simulink model "SympatheticCurrent_Parallel"  (R2015a)
settings: Solver=ode45  StartTime=0.0  StopTime=2  RelTol=1e-4
undefined symbols (not defined in the file or in its folder): D11, Delta
libraries: powerlib x15
settings Model: Creator=baishuhua  LastModifiedBy=baishuhua
settings DebuggingCC: AlgebraicLoopMsg=none

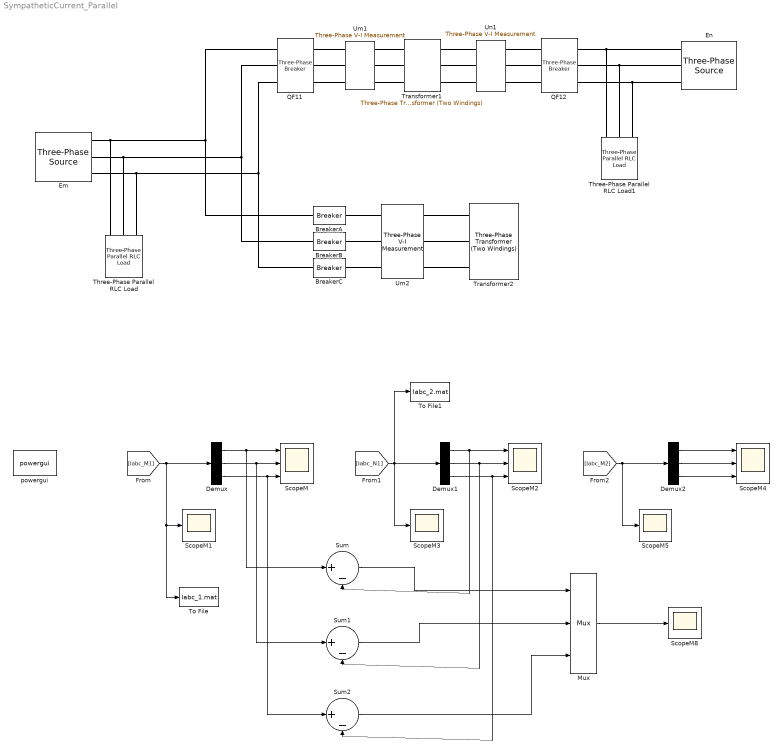
== system SympatheticCurrent_Parallel ==
  BreakerA : powerlib/Elements/Breaker  InitialState=0  SwitchingTimes=[1.1 2]  External=off  BreakerResistance=0.01  SnubberResistance=1e6  SnubberCapacitance=inf  Measurements=None  MoreParameters=on  NoBreakLoop=off
  BreakerB : powerlib/Elements/Breaker  InitialState=0  SwitchingTimes=[1.2 2]  External=off  BreakerResistance=0.01  SnubberResistance=1e6  SnubberCapacitance=inf  Measurements=None  MoreParameters=on  NoBreakLoop=off
  BreakerC : powerlib/Elements/Breaker  InitialState=0  SwitchingTimes=[1.3 2]  External=off  BreakerResistance=0.01  SnubberResistance=1e6  SnubberCapacitance=inf  Measurements=None  MoreParameters=on  NoBreakLoop=off
  Demux : Demux  Outputs=3
  Demux1 : Demux  Outputs=3
  Demux2 : Demux  Outputs=3
  Em : powerlib/Electrical Sources/Three-Phase Source  Voltage=35e3  PhaseAngle=180  Frequency=50  InternalConnection=Yg  SpecifyImpedance=off  Resistance=2.8929  Inductance=16.58e-3  ShortCircuitLevel=100e6  BaseVoltage=35e3  XRratio=7  BusType=swing  Pref=0  Qref=0  Qmin=-inf  Qmax=inf
  En : powerlib/Electrical Sources/Three-Phase Source  Voltage=220e3  PhaseAngle=0  Frequency=50  InternalConnection=Yg  SpecifyImpedance=off  Resistance=0.8929  Inductance=16.58e-3  ShortCircuitLevel=100e6  BaseVoltage=220e3  XRratio=7  BusType=swing  Pref=0  Qref=0  Qmin=-inf  Qmax=inf
  Mux : Mux  Inputs=3
  QF11 : powerlib/Elements/Three-Phase Breaker  InitialState=closed  SwitchA=on  SwitchB=on  SwitchC=on  SwitchTimes="[10  20]"  External=off  BreakerResistance=0.01  SnubberResistance=1e6  SnubberCapacitance=inf  Measurements=None
  QF12 : powerlib/Elements/Three-Phase Breaker  InitialState=open  SwitchA=on  SwitchB=on  SwitchC=on  SwitchTimes=[3 10]  External=off  BreakerResistance=0.01  SnubberResistance=1e6  SnubberCapacitance=inf  Measurements=None
  ScopeM : Scope  NumInputPorts=3
      settings: ShowLegends=on  TimeRange=2  YMin=-500~-4000~-1750  YMax=4000~500~250  SampleInput=on
  ScopeM{1,3,5,8} (4 alike) : Scope
      ScopeM1 settings: ShowLegends=on  TimeRange=5  YMin=-500  YMax=4000  SampleInput=on
      ScopeM3 settings: ShowLegends=on  TimeRange=5  YMin=-500  YMax=4000  SaveName=ScopeData3  SampleInput=on
      ScopeM5 settings: ShowLegends=on  TimeRange=5  YMin=-500  YMax=4000  SaveName=ScopeData5  SampleInput=on
      ScopeM8 settings: ShowLegends=on  TimeRange=5  YMin=-500  YMax=4000  SaveName=ScopeData8  SampleInput=on
  ScopeM2 : Scope  NumInputPorts=3
      settings: ShowLegends=on  TimeRange=1  YMin=-500~-4000~-1750  YMax=4000~500~250  SaveName=ScopeData2  SampleInput=on
  ScopeM4 : Scope  NumInputPorts=3
      settings: ShowLegends=on  TimeRange=10  YMin=-500~-4000~-1750  YMax=4000~500~250  SaveName=ScopeData4  SampleInput=on
  Sum : Sum  Inputs=|+-
  Sum1 : Sum  Inputs=|+-
  Sum2 : Sum  Inputs=|+-
  Three-Phase Parallel RLC Load : powerlib/Elements/Three-Phase Parallel RLC Load  LConnTagsString=A|B|C  Configuration=Y (grounded)  NominalVoltage=35e3  NominalFrequency=50  ActivePower=10e3  InductivePower=100  CapacitivePower=100  Measurements=None  LoadType=constant PQ
  Three-Phase Parallel RLC Load1 : powerlib/Elements/Three-Phase Parallel RLC Load  LConnTagsString=A|B|C  Configuration=Y (grounded)  NominalVoltage=220e3  NominalFrequency=50  ActivePower=10e3  InductivePower=100  CapacitivePower=100  Measurements=None  LoadType=constant PQ
  To File : ToFile  Filename=Iabc_1.mat  MatrixName=Iabc_1  SaveFormat=Timeseries
  To File1 : ToFile  Filename=Iabc_2.mat  MatrixName=Iabc_2  SaveFormat=Timeseries
  Transformer1 : powerlib/Elements/Three-Phase Transformer (Two Windings)  Winding1Connection=Delta (D11)  Winding2Connection=Delta (D11)  CoreType=Three single-phase transformers  SetSaturation=on  Hysteresis=off  DataFile='hysteresis'  SetInitialFlux=on  Measurements=None  UNITS=pu  NominalPower=[ 300e6 , 50 ]  Winding1=[ 35e3 , 0.002 , 0.08 ]  Winding2=[ 220e3 , 0.002 , 0.08 ]  Rm=500  Lm=500  L0=0.5  Saturation=[ 0,0 ; 0.0024,1.2 ; 1.0,1.52 ]  InitialFluxes=[0.5 0 0]  MoreParameters=off  BreakLoop=off  DataType=off  TransfoNumber=1
  Transformer2 : powerlib/Elements/Three-Phase Transformer (Two Windings)  Winding1Connection=Delta (D11)  Winding2Connection=Delta (D11)  CoreType=Three single-phase transformers  SetSaturation=on  Hysteresis=off  DataFile='hysteresis'  SetInitialFlux=on  Measurements=None  UNITS=pu  NominalPower=[ 300e6 , 50 ]  Winding1=[ 35e3 , 0.002 , 0.08 ]  Winding2=[ 220e3 , 0.002 , 0.08 ]  Rm=500  Lm=500  L0=0.5  Saturation=[ 0,0 ; 0.0024,1.2 ; 1.0,1.52 ]  InitialFluxes=[0.7 -0.7 -0.7]  MoreParameters=off  BreakLoop=off  DataType=off  TransfoNumber=1
  Um1 : powerlib/Measurements/Three-Phase V-I Measurement  VoltageMeasurement=no  SetLabelV=on  LabelV=Vabc_M  Vpu=off  VpuLL=off  CurrentMeasurement=yes  SetLabelI=on  LabelI=Iabc_M1  Ipu=on  Pbase=300e6  Vbase=35e3  OutputType=Complex  PhasorSimulation=off  PSBequivalent=0
  Um2 : powerlib/Measurements/Three-Phase V-I Measurement  VoltageMeasurement=no  SetLabelV=on  LabelV=Vabc_M  Vpu=off  VpuLL=off  CurrentMeasurement=yes  SetLabelI=on  LabelI=Iabc_M2  Ipu=on  Pbase=300e6  Vbase=35e3  OutputType=Complex  PhasorSimulation=off  PSBequivalent=0
  Un1 : powerlib/Measurements/Three-Phase V-I Measurement  VoltageMeasurement=no  SetLabelV=on  LabelV=Vabc_N  Vpu=off  VpuLL=off  CurrentMeasurement=yes  SetLabelI=on  LabelI=Iabc_N1  Ipu=on  Pbase=300e6  Vbase=220e3  OutputType=Complex  PhasorSimulation=off  PSBequivalent=0
  powergui : powerlib/powergui  Priority=1  SimulationMode=Discrete  SolverType=Tustin/Backward Euler (TBE)  SampleTime=1e-4  frequency=60  SPID=off  DisableSnubberDevices=off  DisableRonSwitches=off  DisableVfSwitches=off  SwTol=0  DisplayEquations=off  Interpol=off  methode=off  Ts=100  FunctionMessages=off  echomessages=off  HookPort=off  EnableUseOfTLC=off  x0status=blocks  frequencyindice=0  Pbase=100e6  ErrMax=1e-4  Iterations=50  UnitsV=kV  UnitsW=MW  buscounter=0  RestoreLinks=warning  ResistiveCurrentMeasurement=off  Frange=[0:2:500]  Ylog=off  Xlog=on  ShowGrid=off  save=off  variable=ZData  structure=0  ZoomFFT=off  StartTime=0.0  cycles=1  DisplayStyle=1  fundamental=60  FreqAxis=off  MaxFrequency=1000  frequencyindicesteady=1  RmsSteady=1  display=off
  wires:
  [Iabc_M1] -> To File/1, ScopeM1/1, Demux/1
  Demux/1 -> Sum/1, ScopeM/1
  Demux/2 -> ScopeM/2, Sum1/1
  Demux/3 -> ScopeM/3, Sum2/1
  [Iabc_N1] -> To File1/1, ScopeM3/1, Demux1/1
  Demux1/1 -> ScopeM2/1, Sum/2
  Demux1/2 -> ScopeM2/2, Sum1/2
  Demux1/3 -> Sum2/2, ScopeM2/3
  [Iabc_M2] -> ScopeM5/1, Demux2/1
  Demux2/1 -> ScopeM4/1
  Demux2/2 -> ScopeM4/2
  Demux2/3 -> ScopeM4/3
  Sum/1 -> Mux/1
  Sum1/1 -> Mux/2
  Sum2/1 -> Mux/3
  Mux/1 -> ScopeM8/1
  connections:
  Em/RConn1 -- BreakerA/LConn1 -- QF11/LConn1 -- Three-Phase Parallel RLC Load/LConn1
  Em/RConn2 -- BreakerB/LConn1 -- QF11/LConn2 -- Three-Phase Parallel RLC Load/LConn2
  Em/RConn3 -- BreakerC/LConn1 -- QF11/LConn3 -- Three-Phase Parallel RLC Load/LConn3
  QF12/RConn1 -- En/RConn1 -- Three-Phase Parallel RLC Load1/LConn1
  QF12/RConn2 -- En/RConn2 -- Three-Phase Parallel RLC Load1/LConn2
  QF12/RConn3 -- En/RConn3 -- Three-Phase Parallel RLC Load1/LConn3
  Um1/LConn1 -- QF11/RConn1
  Um1/LConn2 -- QF11/RConn2
  Um1/LConn3 -- QF11/RConn3
  Um1/RConn1 -- Transformer1/LConn1
  Um1/RConn2 -- Transformer1/LConn2
  Um1/RConn3 -- Transformer1/LConn3
  Un1/LConn1 -- Transformer1/RConn1
  Un1/LConn2 -- Transformer1/RConn2
  Un1/LConn3 -- Transformer1/RConn3
  Un1/RConn1 -- QF12/LConn1
  Un1/RConn2 -- QF12/LConn2
  Un1/RConn3 -- QF12/LConn3
  BreakerA/RConn1 -- Um2/LConn1
  BreakerB/RConn1 -- Um2/LConn2
  BreakerC/RConn1 -- Um2/LConn3
  Um2/RConn1 -- Transformer2/LConn1
  Um2/RConn2 -- Transformer2/LConn2
  Um2/RConn3 -- Transformer2/LConn3
